simulink model "quadcopter_model"  (R2024a)
settings: Solver=ode4  StartTime=0.0  StopTime=300  FixedStep=0.001  RelTol=1e-10  AbsTol=1e-10
values from neighbouring files (symbols this model uses):
  a1 = 7.6923e-4    (= 0.00076923)    [quadcopter_param.m]    (also in satellite_param.m = ab1 / I(1,1); unicycle_param.m = 4e-05)
  a2 = 1e-3    (= 0.001)    [quadcopter_param.m]    (also in satellite_param.m = ab2 / I(2,2); unicycle_param.m = 0.0052)
  a3 = 6.5385e-4    (= 0.00065385)    [quadcopter_param.m]    (also in satellite_param.m = ab3 / I(3,3))
  c1 = 20.5333    [quadcopter_param.m]    (also in satellite_param.m = cb1 / I(1,1); unicycle_param.m = 0.4)
  c2 = 31.6    [quadcopter_param.m]    (also in satellite_param.m = cb2 / I(2,2); unicycle_param.m = 2.4)
  c3 = 14.2308    [quadcopter_param.m]    (also in satellite_param.m = cb3 / I(3,3))
  delay = 0.01    [quadcopter_param.m]    (also in satellite_param.m = 0.003; unicycle_param.m)
  k = 3.95    [quadcopter_param.m]    (also in satellite_param.m = 2.4; unicycle_param.m = 12.5)
  omega = 25    [quadcopter_param.m]    (also in satellite_param.m = 36; unicycle_param.m = 50)
  variance = 1e-6    (= 1e-06)    [quadcopter_param.m]    (also in satellite_param.m = 1e-09; unicycle_param.m)
settings Model: Creator=rohan  LastModifiedBy=rohan

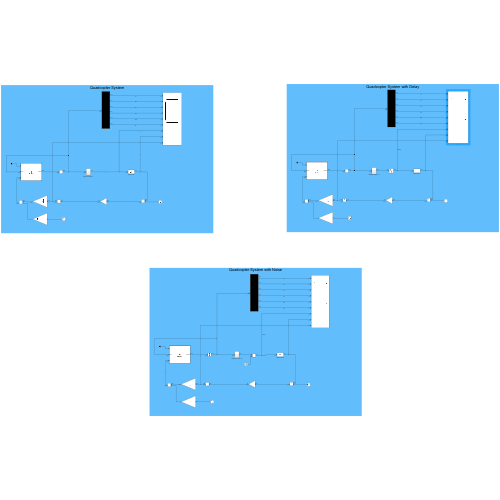
[thumbnail: Simulink's stored preview of the top-level diagram]
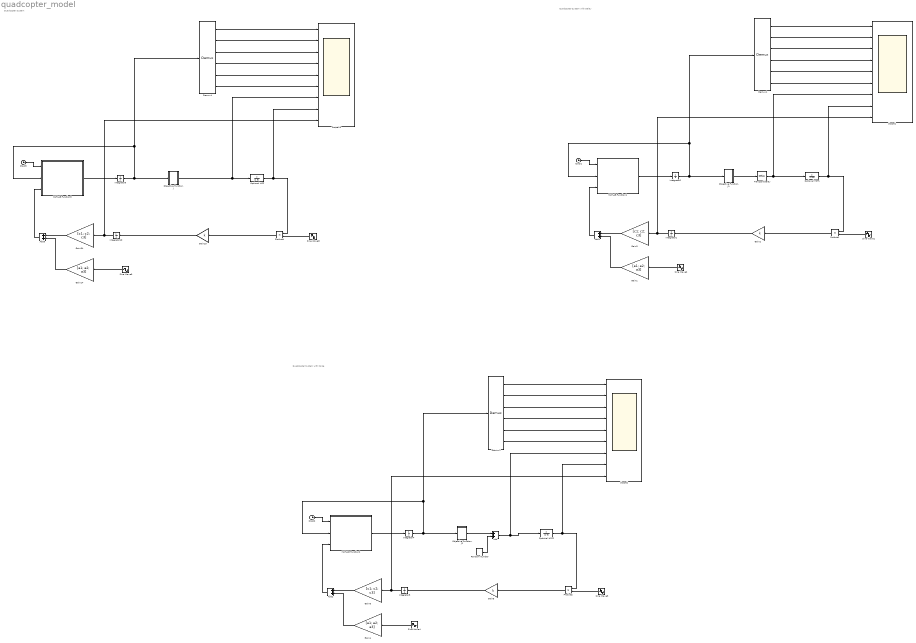
== system quadcopter_model ==
  note: Quadcopter System
  note: Quadcopter System with Delay
  note: Quadcopter System with Noise
  Add{,1..2,5} (4 alike) : Sum
  Clock1 : Clock
  Clock2 : Clock
  Clock5 : Clock
  Demux1 : Demux  Outputs=6
  Demux2 : Demux  Outputs=6
  Demux4 : Demux  Outputs=6
  Gain1 : Gain  Gain=[a1; a2; a3]
  Gain14 : Gain  Gain=[a1; a2; a3]
  Gain15 : Gain  Gain=k
  Gain2 : Gain  Gain=k
  Gain3 : Gain  Gain=[c1; c2; c3]
  Gain34 : Gain  Gain=[c1; c2; c3]
  Gain4 : Gain  Gain=[a1; a2; a3]
  Gain5 : Gain  Gain=k
  Gain6 : Gain  Gain=[c1; c2; c3]
  Integrator1 : Integrator
  Integrator10 : Integrator
  Integrator2 : Integrator  InitialCondition=[0; 0; 0; 10*pi/180; 15*pi/180; 12*pi/180]
  Integrator3 : Integrator
  Integrator4 : Integrator  InitialCondition=[0; 0; 0; 10*pi/180; 15*pi/180; 12*pi/180]
  Integrator9 : Integrator  InitialCondition=[0; 0; 0; 10*pi/180; 15*pi/180; 12*pi/180]
  MATLAB Function1 : MATLAB Function  TreatAsAtomicUnit=on
  MATLAB Function2 : MATLAB Function  TreatAsAtomicUnit=on
  MATLAB Function5 : MATLAB Function  TreatAsAtomicUnit=on
  "Objective Function, J" : Subsystem
  "Objective Function, J1" : Subsystem
  "Objective Function, J2" : Subsystem
  Optional HPF : TransferFcn  Numerator=[1 0]  Denominator=[1 e]
  Optional HPF1 : TransferFcn  Numerator=[1 0]  Denominator=[1 e]
  Optional HPF2 : TransferFcn  Numerator=[1 0]  Denominator=[1 e]
  Product1 : Product
  Product2 : Product
  Product4 : Product
  Random Number : RandomNumber  Variance=variance  Seed=1  SampleTime=0.001
  Scope1 : Scope  NumInputPorts=9
  Scope13 : Scope  NumInputPorts=9
  Scope2 : Scope  NumInputPorts=9
  Sine Wave{1..4,8..9} (6 alike) : Sin  Amplitude=omega  Frequency=omega  Phase=pi/2  SampleTime=0
  Transport Delay : TransportDelay  DelayTime=delay  InitialOutput=(10*pi/180 - 0)^2 + (15*pi/180 - 0)^2 + (12*pi/180 - 0)^2
  wires:
  Optional HPF/1 -> Product4/1, Scope13/8  "h"
  Demux4/4 -> Scope13/4  "psi"
  Product4/1 -> Gain15/1
  Gain15/1 -> Integrator10/1  "lpf"
  Demux4/2 -> Scope13/2  "w2"
  Demux4/5 -> Scope13/5  "theta"
  Integrator9/1 -> "Objective Function, J"/1(In1), MATLAB Function5/2(state), Demux4/1
  Gain14/1 -> Add5/2
  Demux4/1 -> Scope13/1  "w1"
  Demux4/3 -> Scope13/3  "w3"
  Add5/1 -> MATLAB Function5/3(u)  "u"
  Demux4/6 -> Scope13/6  "phi"
  Sine Wave8/1 -> Product4/2
  MATLAB Function5/1(statedot) -> Integrator9/1
  Sine Wave9/1 -> Gain14/1
  Clock5/1 -> MATLAB Function5/1(t)
  "Objective Function, J"/1(Out1) -> Optional HPF/1, Scope13/7  "J"
  Integrator10/1 -> Scope13/9, Gain34/1  "uhat"
  Gain34/1 -> Add5/1
  Gain1/1 -> Add1/2
  Gain3/1 -> Add1/1
  Add1/1 -> MATLAB Function1/3(u)  "u"
  Clock1/1 -> MATLAB Function1/1(t)
  Demux1/2 -> Scope1/2  "w2"
  MATLAB Function1/1(statedot) -> Integrator2/1
  Demux1/6 -> Scope1/6  "phi"
  Demux1/1 -> Scope1/1  "w1"
  Demux1/4 -> Scope1/4  "psi"
  Optional HPF1/1 -> Product1/1, Scope1/8  "h"
  Product1/1 -> Gain2/1
  Gain2/1 -> Integrator1/1  "lpf"
  Sine Wave2/1 -> Gain1/1
  Demux1/5 -> Scope1/5  "theta"
  Integrator2/1 -> "Objective Function, J1"/1(In1), MATLAB Function1/2(state), Demux1/1
  Sine Wave1/1 -> Product1/2
  "Objective Function, J1"/1(Out1) -> Transport Delay/1  "J"
  Demux1/3 -> Scope1/3  "w3"
  Integrator1/1 -> Scope1/9, Gain3/1  "uhat"
  Transport Delay/1 -> Scope1/7, Optional HPF1/1  "J+delay"
  Integrator3/1 -> Scope2/9, Gain6/1  "uhat"
  Demux2/3 -> Scope2/3  "w3"
  "Objective Function, J2"/1(Out1) -> Add/1  "J"
  Integrator4/1 -> "Objective Function, J2"/1(In1), MATLAB Function2/2(state), Demux2/1
  Sine Wave4/1 -> Gain4/1
  Gain5/1 -> Integrator3/1  "lpf"
  Demux2/5 -> Scope2/5  "theta"
  Optional HPF2/1 -> Product2/1, Scope2/8  "h"
  Product2/1 -> Gain5/1
  Demux2/6 -> Scope2/6  "phi"
  Sine Wave3/1 -> Product2/2
  Add/1 -> Scope2/7, Optional HPF2/1  "J+noise"
  MATLAB Function2/1(statedot) -> Integrator4/1
  Demux2/1 -> Scope2/1  "w1"
  Gain4/1 -> Add2/2
  Demux2/2 -> Scope2/2  "w2"
  Gain6/1 -> Add2/1
  Clock2/1 -> MATLAB Function2/1(t)
  Demux2/4 -> Scope2/4  "psi"
  Add2/1 -> MATLAB Function2/3(u)  "u"
  Random Number/1 -> Add/2

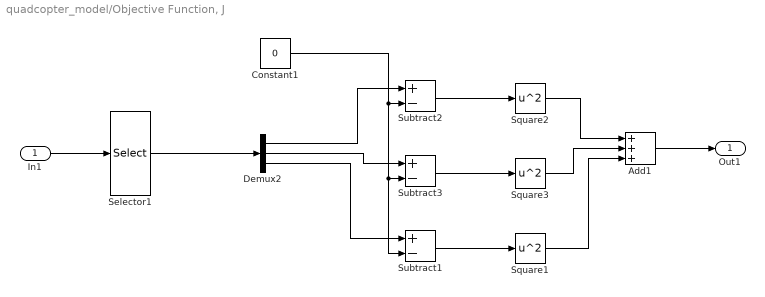
== system quadcopter_model/Objective Function, J ==
  In1 : Inport
  Add1 : Sum  Inputs=+++
  Constant1 : Constant  Value=0
  Demux2 : Demux  Outputs=3
  Selector1 : Selector  InputPortWidth=6  IndexOptions=Index vector (dialog)  Indices=[4 5 6]  OutputSizes=1
  Square1 : Math  Operator=square
  Square2 : Math  Operator=square
  Square3 : Math  Operator=square
  Subtract1 : Sum  Inputs=+-
  Subtract2 : Sum  Inputs=+-
  Subtract3 : Sum  Inputs=+-
  Out1 : Outport
  wires:
  Demux2/1 -> Subtract2/1
  Selector1/1 -> Demux2/1
  Constant1/1 -> Subtract1/2, Subtract3/2, Subtract2/2
  Square2/1 -> Add1/1
  Square3/1 -> Add1/2
  Demux2/2 -> Subtract3/1
  Subtract3/1 -> Square3/1
  Subtract2/1 -> Square2/1
  Add1/1 -> Out1/1
  In1/1 -> Selector1/1
  Demux2/3 -> Subtract1/1
  Subtract1/1 -> Square1/1
  Square1/1 -> Add1/3

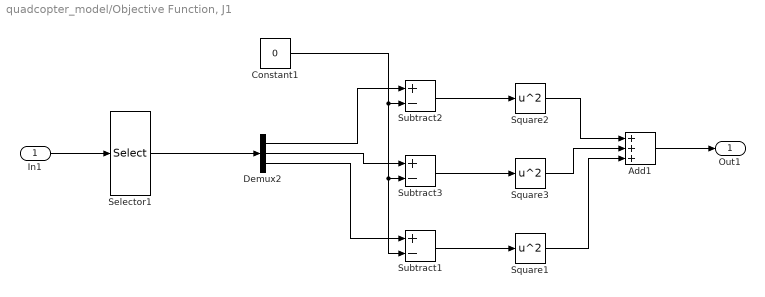
== system quadcopter_model/Objective Function, J1 ==
  In1 : Inport
  Add1 : Sum  Inputs=+++
  Constant1 : Constant  Value=0
  Demux2 : Demux  Outputs=3
  Selector1 : Selector  InputPortWidth=6  IndexOptions=Index vector (dialog)  Indices=[4 5 6]  OutputSizes=1
  Square1 : Math  Operator=square
  Square2 : Math  Operator=square
  Square3 : Math  Operator=square
  Subtract1 : Sum  Inputs=+-
  Subtract2 : Sum  Inputs=+-
  Subtract3 : Sum  Inputs=+-
  Out1 : Outport
  wires:
  Demux2/1 -> Subtract2/1
  Selector1/1 -> Demux2/1
  Constant1/1 -> Subtract1/2, Subtract3/2, Subtract2/2
  Square2/1 -> Add1/1
  Square3/1 -> Add1/2
  Demux2/2 -> Subtract3/1
  Subtract3/1 -> Square3/1
  Subtract2/1 -> Square2/1
  Add1/1 -> Out1/1
  In1/1 -> Selector1/1
  Demux2/3 -> Subtract1/1
  Subtract1/1 -> Square1/1
  Square1/1 -> Add1/3

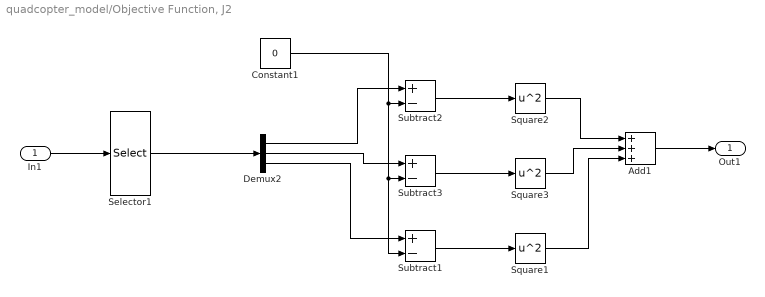
== system quadcopter_model/Objective Function, J2 ==
  In1 : Inport
  Add1 : Sum  Inputs=+++
  Constant1 : Constant  Value=0
  Demux2 : Demux  Outputs=3
  Selector1 : Selector  InputPortWidth=6  IndexOptions=Index vector (dialog)  Indices=[4 5 6]  OutputSizes=1
  Square1 : Math  Operator=square
  Square2 : Math  Operator=square
  Square3 : Math  Operator=square
  Subtract1 : Sum  Inputs=+-
  Subtract2 : Sum  Inputs=+-
  Subtract3 : Sum  Inputs=+-
  Out1 : Outport
  wires:
  Demux2/1 -> Subtract2/1
  Selector1/1 -> Demux2/1
  Constant1/1 -> Subtract1/2, Subtract3/2, Subtract2/2
  Square2/1 -> Add1/1
  Square3/1 -> Add1/2
  Demux2/2 -> Subtract3/1
  Subtract3/1 -> Square3/1
  Subtract2/1 -> Square2/1
  Add1/1 -> Out1/1
  In1/1 -> Selector1/1
  Demux2/3 -> Subtract1/1
  Subtract1/1 -> Square1/1
  Square1/1 -> Add1/3

== matlab function quadcopter_model/MATLAB Function2 ==
  data: t input; state input; u input; statedot output
function statedot = dynamics(t,state,u)
w1 = state(1);
w2 = state(2);
w3 = state(3);
psi = state(4);
theta = state(5);
phi = state(6);

kr = diag([0.1, 0.1, 0.15]);
I = diag([0.0075, 0.0075, 0.013]); % kg*m^2

wArray = [w1; w2; w3];
wSkewSym = [0 -w3 w2;
            w3 0 -w1;
            -w2 w1 0];


wdot = I\(-wSkewSym*(I*wArray) - kr*wArray) + u;

angdot = ((1/cos(theta)) .* [0, sin(phi), cos(phi);
                            0, cos(phi)*cos(theta), -sin(phi)*cos(theta);
                            cos(theta), sin(phi)*sin(theta), cos(phi)*sin(theta)]) * wArray;


statedot = [wdot; angdot];
end

== matlab function quadcopter_model/MATLAB Function5 ==
  data: t input; state input; u input; statedot output
function statedot = dynamics(t,state,u)
w1 = state(1);
w2 = state(2);
w3 = state(3);
psi = state(4);
theta = state(5);
phi = state(6);

kr = diag([0.1, 0.1, 0.15]);
I = diag([0.0075, 0.0075, 0.013]); % kg*m^2

wArray = [w1; w2; w3];
wSkewSym = [0 -w3 w2;
            w3 0 -w1;
            -w2 w1 0];


wdot = I\(-wSkewSym*(I*wArray) - kr*wArray) + u;

angdot = ((1/cos(theta)) .* [0, sin(phi), cos(phi);
                            0, cos(phi)*cos(theta), -sin(phi)*cos(theta);
                            cos(theta), sin(phi)*sin(theta), cos(phi)*sin(theta)]) * wArray;


statedot = [wdot; angdot];
end

== matlab function quadcopter_model/MATLAB Function1 ==
  data: t input; state input; u input; statedot output
function statedot = dynamics(t,state,u)
w1 = state(1);
w2 = state(2);
w3 = state(3);
psi = state(4);
theta = state(5);
phi = state(6);

kr = diag([0.1, 0.1, 0.15]);
I = diag([0.0075, 0.0075, 0.013]); % kg*m^2

wArray = [w1; w2; w3];
wSkewSym = [0 -w3 w2;
            w3 0 -w1;
            -w2 w1 0];


wdot = I\(-wSkewSym*(I*wArray) - kr*wArray) + u;

angdot = ((1/cos(theta)) .* [0, sin(phi), cos(phi);
                            0, cos(phi)*cos(theta), -sin(phi)*cos(theta);
                            cos(theta), sin(phi)*sin(theta), cos(phi)*sin(theta)]) * wArray;


statedot = [wdot; angdot];
end
